simulink model "lab3_0x2820x29"  (R2024a)
settings: Solver=VariableStepAuto  StartTime=0.0  StopTime=0.05  RelTol=1e-3
undefined symbols (not defined in the file): magnitude
libraries: dspstat3 x5, dspfdesign x3, commsynccomp2 x1, spspowerguiLib x1
settings Model: Creator=CS Net Games  LastModifiedBy=hp
settings SolverCC: AlgebraicLoopSolver=TrustRegion
settings DebuggingCC: UnconnectedInputMsg=warning  UnconnectedOutputMsg=warning  UnconnectedLineMsg=warning
settings ModelReferenceCC: EnableRefExpFcnMdlSchedulingChecks=on
settings SFSimCC: CustomCodeUndefinedFunction=UseInterfaceOnly
settings RTWCC: GPUComputeCapability=3.5

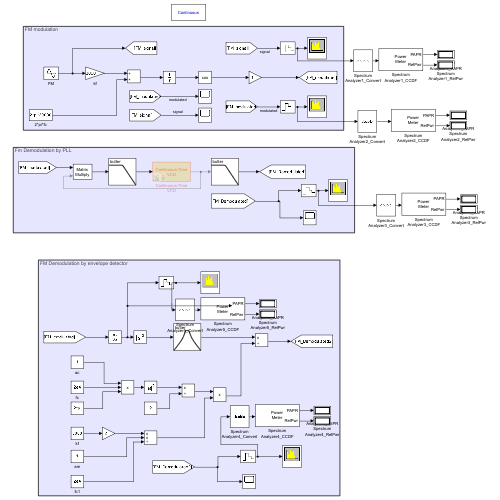
[thumbnail: Simulink's stored preview of the top-level diagram]
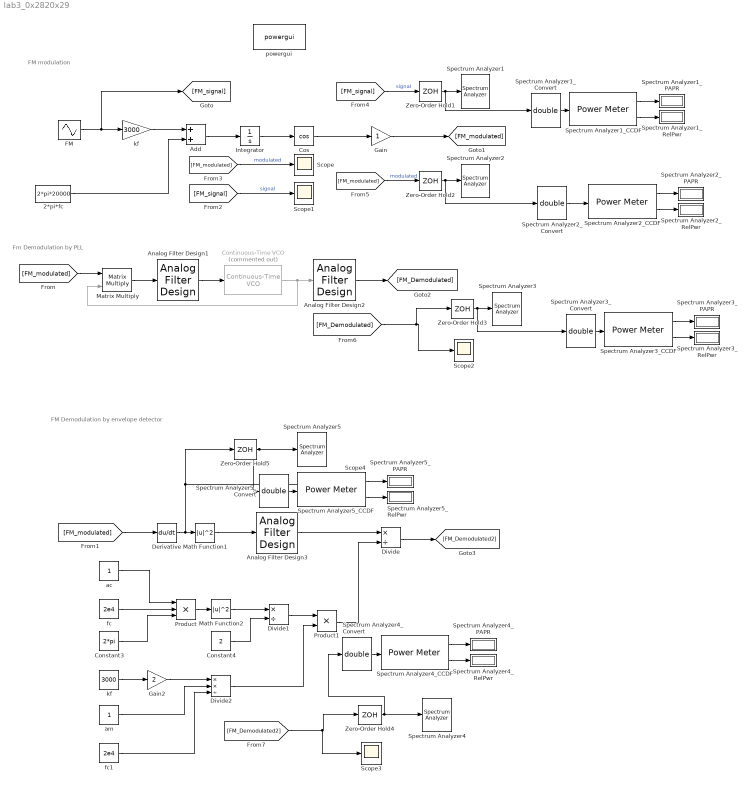
== system lab3_0x2820x29 ==
  note: FM Demodulation by envelope detector
  note: Fm Demodulation by PLL
  note: FM modulation
  2*pi*fc : Constant  Value=2*pi*20000
  Add : Sum
  Analog Filter Design1 : dspfdesign/Analog Filter Design  method=Butterworth  filttype=Lowpass  N=8  Wlo=2*pi*600  Whi=80  Rp=2  Rs=40
  Analog Filter Design2 : dspfdesign/Analog Filter Design  method=Butterworth  filttype=Lowpass  N=8  Wlo=pi*2*600  Whi=80  Rp=2  Rs=40
  Analog Filter Design3 : dspfdesign/Analog Filter Design  method=Butterworth  filttype=Bandpass  N=8  Wlo=400*2*pi  Whi=700*2*pi  Rp=2  Rs=40
  Constant3 : Constant  Value=2*pi
  Constant4 : Constant  Value=2
  Continuous-Time VCO : commsynccomp2/Continuous-Time VCO  Commented=on  Ac=1  Fc=500  Kc=1  Ph=0
  Cos : Trigonometry  Operator=cos
  Derivative : Derivative
  Divide : Product  Inputs=*/
  Divide1 : Product  Inputs=*/
  Divide2 : Product  Inputs=**/
  "FM " : Sin  Frequency=pi*2*500  SampleTime=0
  Gain : Gain
  Gain2 : Gain  Gain=2
  Integrator : Integrator
  Math Function1 : Math  Operator=magnitude^2  SignedPower=on
  Math Function2 : Math  Operator=magnitude^2  SignedPower=on
  Matrix Multiply : Product  Multiplication=Matrix(*)
  Product : Product  Inputs=3
  Product1 : Product
  Scope{,1..4} (5 alike) : Scope
  Spectrum Analyzer1 : SpectrumAnalyzer  WindowPosition=[-6.000000,-9.000000,1282.000000,700.000000,]  ScopeFrameLocation=window  SpectrumType=RMS  Method=Welch  SampleRate=5000  AxesScaling=Manual  AveragingMethod=Running  SpectrumUnits=Vrms  YLimits=[-0.060904247557560707571,0.54813822882120266655]  ShowLegend=on  ChannelNames="[\"FM message signal\"]"  AllowFFTLengthLessThanSamplesPerUpdate=on  DefaultConfigurationName=spbscopes.SpectrumAnalyzerBlockCfg  IsFrequencyInputMode=0  FrequencyVectorPort=0  FrequencyVectorFromPort=0  FrequencyInputRBWPort=0  FrequencyInputRBWFromPort=0
      settings: OpenAtSimulationStart=off
  Spectrum Analyzer1_CCDF : dspstat3/Power Meter  Measurement=Peak-to-average power ratio  ReferenceLoad=1  OutputPowerUnits=dBm  WindowLength=256  OverlapLength=255  AllowArbitraryInputLength=off  ComputeCCDF=on  PowerRange=50  PowerResolution=0.1  CCDFOutput=Relative power (dB above average power)  ProbabilityVector=[ 10; 1; 0.1; 0.01; 0.001; 0.0001 ]  RelativePowerVector=[ 0; 3; 6; 9; 12 ]  ResetPort=off  SimulateUsing=Interpreted execution
  Spectrum Analyzer1_Convert : DataTypeConversion  OutDataTypeStr=double
  Spectrum Analyzer1_PAPR : Display
  Spectrum Analyzer1_RelPwr : Display
  Spectrum Analyzer2 : SpectrumAnalyzer  WindowPosition=[-128.000000,-14.000000,1282.000000,700.000000,]  ScopeFrameLocation=window  SpectrumType=RMS  Method=Welch  SampleRate=200000  AxesScaling=Manual  AveragingMethod=Running  SpectrumUnits=Vrms  YLimits=[-0.044331986242742905946,0.39898787640275168442]  ShowLegend=on  ChannelNames="[\"Fm modulated signal\"]"  AllowFFTLengthLessThanSamplesPerUpdate=on  DefaultConfigurationName=spbscopes.SpectrumAnalyzerBlockCfg  IsFrequencyInputMode=0  FrequencyVectorPort=0  FrequencyVectorFromPort=0  FrequencyInputRBWPort=0  FrequencyInputRBWFromPort=0
      settings: OpenAtSimulationStart=off
  Spectrum Analyzer2_CCDF : dspstat3/Power Meter  Measurement=Peak-to-average power ratio  ReferenceLoad=1  OutputPowerUnits=dBm  WindowLength=256  OverlapLength=255  AllowArbitraryInputLength=off  ComputeCCDF=on  PowerRange=50  PowerResolution=0.1  CCDFOutput=Relative power (dB above average power)  ProbabilityVector=[ 10; 1; 0.1; 0.01; 0.001; 0.0001 ]  RelativePowerVector=[ 0; 3; 6; 9; 12 ]  ResetPort=off  SimulateUsing=Interpreted execution
  Spectrum Analyzer2_Convert : DataTypeConversion  OutDataTypeStr=double
  Spectrum Analyzer2_PAPR : Display
  Spectrum Analyzer2_RelPwr : Display
  Spectrum Analyzer3 : SpectrumAnalyzer  WindowPosition=[-128.000000,-14.000000,1282.000000,700.000000,]  Visible=on  ScopeFrameLocation=window  SpectrumType=RMS  Method=Welch  SampleRate=5000  AxesScaling=Manual  AveragingMethod=Running  SpectrumUnits=Vrms  YLimits=[-0.062357931574312124023,0.56122138431727885965]  ShowLegend=on  ChannelNames="[\"demodulation using PLL\"]"  AllowFFTLengthLessThanSamplesPerUpdate=on  DefaultConfigurationName=spbscopes.SpectrumAnalyzerBlockCfg  IsFrequencyInputMode=0  FrequencyVectorPort=0  FrequencyVectorFromPort=0  FrequencyInputRBWPort=0  FrequencyInputRBWFromPort=0
      settings: OpenAtSimulationStart=off
  Spectrum Analyzer3_CCDF : dspstat3/Power Meter  Measurement=Peak-to-average power ratio  ReferenceLoad=1  OutputPowerUnits=dBm  WindowLength=256  OverlapLength=255  AllowArbitraryInputLength=off  ComputeCCDF=on  PowerRange=50  PowerResolution=0.1  CCDFOutput=Relative power (dB above average power)  ProbabilityVector=[ 10; 1; 0.1; 0.01; 0.001; 0.0001 ]  RelativePowerVector=[ 0; 3; 6; 9; 12 ]  ResetPort=off  SimulateUsing=Interpreted execution
  Spectrum Analyzer3_Convert : DataTypeConversion  OutDataTypeStr=double
  Spectrum Analyzer3_PAPR : Display
  Spectrum Analyzer3_RelPwr : Display
  Spectrum Analyzer4 : SpectrumAnalyzer  WindowPosition=[-1.000000,10.000000,1282.000000,700.000000,]  ScopeFrameLocation=window  SpectrumType=RMS  Method=Welch  SampleRate=5000  AxesScaling=Manual  AveragingMethod=Running  SpectrumUnits=Vrms  YLimits=[-0.0088911251986494369004,0.0800201267902619362]  ShowLegend=on  ChannelNames="[\"FM Demodulation by envelope detector\"]"  SelectedToolstripTab=spectrumAnalyzerToolstrip.estimationTab  AllowFFTLengthLessThanSamplesPerUpdate=on  DefaultConfigurationName=spbscopes.SpectrumAnalyzerBlockCfg  IsFrequencyInputMode=0  FrequencyVectorPort=0  FrequencyVectorFromPort=0  FrequencyInputRBWPort=0  FrequencyInputRBWFromPort=0
      settings: OpenAtSimulationStart=off
  Spectrum Analyzer4_CCDF : dspstat3/Power Meter  Measurement=Peak-to-average power ratio  ReferenceLoad=1  OutputPowerUnits=dBm  WindowLength=256  OverlapLength=255  AllowArbitraryInputLength=off  ComputeCCDF=on  PowerRange=50  PowerResolution=0.1  CCDFOutput=Relative power (dB above average power)  ProbabilityVector=[ 10; 1; 0.1; 0.01; 0.001; 0.0001 ]  RelativePowerVector=[ 0; 3; 6; 9; 12 ]  ResetPort=off  SimulateUsing=Interpreted execution
  Spectrum Analyzer4_Convert : DataTypeConversion  OutDataTypeStr=double
  Spectrum Analyzer4_PAPR : Display
  Spectrum Analyzer4_RelPwr : Display
  Spectrum Analyzer5 : SpectrumAnalyzer  WindowPosition=[1.000000,1.000000,1280.000000,697.000000,]  ScopeFrameLocation=window  SpectrumType=RMS  Method=Welch  SampleRate=200000  AxesScaling=Manual  AveragingMethod=Running  SpectrumUnits=Vrms  YLimits=[-5580.1735660495241973,50269.691680596522929]  ShowLegend=on  ChannelNames="[\"frequency for ds/dt for modulated signal\"]"  AllowFFTLengthLessThanSamplesPerUpdate=on  DefaultConfigurationName=spbscopes.SpectrumAnalyzerBlockCfg  IsFrequencyInputMode=0  FrequencyVectorPort=0  FrequencyVectorFromPort=0  FrequencyInputRBWPort=0  FrequencyInputRBWFromPort=0
      settings: OpenAtSimulationStart=off
  Spectrum Analyzer5_CCDF : dspstat3/Power Meter  Measurement=Peak-to-average power ratio  ReferenceLoad=1  OutputPowerUnits=dBm  WindowLength=256  OverlapLength=255  AllowArbitraryInputLength=off  ComputeCCDF=on  PowerRange=50  PowerResolution=0.1  CCDFOutput=Relative power (dB above average power)  ProbabilityVector=[ 10; 1; 0.1; 0.01; 0.001; 0.0001 ]  RelativePowerVector=[ 0; 3; 6; 9; 12 ]  ResetPort=off  SimulateUsing=Interpreted execution
  Spectrum Analyzer5_Convert : DataTypeConversion  OutDataTypeStr=double
  Spectrum Analyzer5_PAPR : Display
  Spectrum Analyzer5_RelPwr : Display
  Zero-Order Hold1 : ZeroOrderHold  SampleTime=1/(10*5e2)
  Zero-Order Hold2 : ZeroOrderHold  SampleTime=1/(10*2e4)
  Zero-Order Hold3 : ZeroOrderHold  SampleTime=1/(10*500)
  Zero-Order Hold4 : ZeroOrderHold  SampleTime=1/(10*500)
  Zero-Order Hold5 : ZeroOrderHold  SampleTime=-1
  ac : Constant
  "am " : Constant
  fc : Constant  Value=2e4
  fc1 : Constant  Value=2e4
  kf : Gain  Gain=3000
  "kf " : Constant  Value=3000
  powergui : spspowerguiLib/powergui  Priority=1  SimulationMode=Continuous  SampleTime=50e-6  frequency=60  Iterations=50  frequencyindice=60  Pbase=100e6  ErrMax=1e-4  UnitsV=kV  UnitsW=MW  buscounter=0  FunctionMessages=off  echomessages=off  EnableUseOfTLC=off  CurrentSourceSwitches=off  DisableSnubberDevices=off  DisableRonSwitches=off  DisableVfSwitches=off  DisplayEquations=off  AutomaticDiscreteSolvers=off  SolverType=Tustin/Backward Euler (TBE)  Interpol=off  ExternalGateDelay=off  methode=off  Ts=100  x0status=blocks  SPID=on  SwTol=0  HookPort=off  NonlinearTolerance=0  nMaxIteration=15  ContinueOnMaxIteration=off  RestoreLinks=warning  ResistiveCurrentMeasurement=off  Frange=[0:2:500]  Ylog=off  Xlog=on  ShowGrid=off  save=off  variable=ZData  structure=0  ZoomFFT=off  StartTime=0.0  cycles=1  DisplayStyle=1  fundamental=60  FreqAxis=off  MaxFrequency=1000  frequencyindicesteady=1  RmsSteady=1  display=off
  wires:
  [FM_modulated] -> Scope/1  "modulated"
  Add/1 -> Integrator/1
  [FM_signal] -> Scope1/1  "signal"
  Zero-Order Hold2/1 -> Spectrum Analyzer2/1, Spectrum Analyzer2_Convert/1
  Zero-Order Hold1/1 -> Spectrum Analyzer1/1, Spectrum Analyzer1_Convert/1
  kf/1 -> Add/1
  Integrator/1 -> Cos/1
  Cos/1 -> Gain/1
  "FM "/1 -> [FM_signal], kf/1
  Gain/1 -> [FM_modulated]
  [FM_signal] -> Zero-Order Hold1/1  "signal"
  2*pi*fc/1 -> Add/2
  [FM_modulated] -> Zero-Order Hold2/1  "modulated"
  Zero-Order Hold3/1 -> Spectrum Analyzer3/1, Spectrum Analyzer3_Convert/1
  [FM_Demodulated] -> Scope2/1, Zero-Order Hold3/1
  Analog Filter Design1/1 -> Continuous-Time VCO/1
  Analog Filter Design2/1 -> [FM_Demodulated]
  [FM_modulated] -> Matrix Multiply/1
  Continuous-Time VCO/1 -> Matrix Multiply/2, Analog Filter Design2/1
  Matrix Multiply/1 -> Analog Filter Design1/1
  Divide/1 -> [FM_Demodulated2]
  Zero-Order Hold5/1 -> Spectrum Analyzer5/1, Spectrum Analyzer5_Convert/1
  fc/1 -> Product/2
  Zero-Order Hold4/1 -> Spectrum Analyzer4/1, Spectrum Analyzer4_Convert/1
  Analog Filter Design3/1 -> Divide/1
  Product/1 -> Math Function2/1
  Divide1/1 -> Product1/1
  [FM_Demodulated2] -> Scope3/1, Zero-Order Hold4/1
  Divide2/1 -> Product1/2
  "am "/1 -> Divide2/2
  Product1/1 -> Divide/2
  fc1/1 -> Divide2/3
  Derivative/1 -> Zero-Order Hold5/1, Scope4/1, Math Function1/1
  [FM_modulated] -> Derivative/1
  Math Function1/1 -> Analog Filter Design3/1
  Constant3/1 -> Product/3
  "kf "/1 -> Gain2/1
  Math Function2/1 -> Divide1/1
  Gain2/1 -> Divide2/1
  Constant4/1 -> Divide1/2
  ac/1 -> Product/1
  Spectrum Analyzer3_Convert/1 -> Spectrum Analyzer3_CCDF/1
  Spectrum Analyzer3_CCDF/1 -> Spectrum Analyzer3_PAPR/1
  Spectrum Analyzer3_CCDF/2 -> Spectrum Analyzer3_RelPwr/1
  Spectrum Analyzer4_Convert/1 -> Spectrum Analyzer4_CCDF/1
  Spectrum Analyzer4_CCDF/1 -> Spectrum Analyzer4_PAPR/1
  Spectrum Analyzer4_CCDF/2 -> Spectrum Analyzer4_RelPwr/1
  Spectrum Analyzer1_Convert/1 -> Spectrum Analyzer1_CCDF/1
  Spectrum Analyzer1_CCDF/1 -> Spectrum Analyzer1_PAPR/1
  Spectrum Analyzer1_CCDF/2 -> Spectrum Analyzer1_RelPwr/1
  Spectrum Analyzer5_Convert/1 -> Spectrum Analyzer5_CCDF/1
  Spectrum Analyzer5_CCDF/1 -> Spectrum Analyzer5_PAPR/1
  Spectrum Analyzer5_CCDF/2 -> Spectrum Analyzer5_RelPwr/1
  Spectrum Analyzer2_Convert/1 -> Spectrum Analyzer2_CCDF/1
  Spectrum Analyzer2_CCDF/1 -> Spectrum Analyzer2_PAPR/1
  Spectrum Analyzer2_CCDF/2 -> Spectrum Analyzer2_RelPwr/1
